simulink model "INTEGRATION_TEST_01"  (Simulink 8.1)
settings: Solver=ode4  StartTime=0.0  StopTime=inf  FixedStep=Ts  MaxStep=1e-3  RelTol=1e-3
PostLoadFcn:
  | INTEGRATION_TEST_01_init;
InitFcn:
  | INTEGRATION_TEST_01_init;
values from neighbouring files (symbols this model uses):
  CMD_signals = [1 2 3 4 5 6 7 8 9 10 11 12 ... (1568 elements, 49x32)]    [CMD_signals.mat]    (also in TestProcedure_xlsRead.m = [time_vec POI_all diesel solarIrr solarBreaker CHP load_gain)
  SIM_HIL = 0    [INTEGRATION_TEST_01_init.m]
  Ts = 100E-6    (= 0.0001)    [INTEGRATION_TEST_01_init.m]
undefined symbols (not defined in the file or in its folder): cable_spec, fdesignblkfcn, gcbh, Left, NG_CHP, NG_CHP_lib, ph, relay_par, type, V
libraries: simulink x23, rtio_opalrt_common x21, rtlab x7, powerlib_extras x7, simulink_extras x7, cables_lib x6, breaker_lib x4, rtio_generic_modbus x4, rteventslib x4, Load_lib x3, powerlib x2, ssn_lib x2
(part 3 of 3)

== matlab function SM_system/Scheduler ==
  data: u input double; y output double; CMD_signals input double; n input double; n1 output double
function [y,n1] = fcn(u,CMD_signals,n)
% Author: Matthew Backes, MIT Lincoln Laboratory
% Date: 8/16/2016
%
% Edited 9/6/2016 by E. Corbett to remove repeated Modbus register 0007 for
% DSO Import value
%
% This function takes in the test sequence signals from a .mat file which
% is generated with the ____.m script. It then updates the parameters
% within the simulink model according to the time stamp of the test
% sequence command signals.
% CMD column 1 = time
% CMD column 2 = POI feeder 1 SEL relay
% CMD column 3 = POI feeder 2 SEL relay
% CMD column 4 = POI feeder 3 SEL relay
% CMD column 5 = diesel breaker
% CMD column 6 = solar irradiance gain
% CMD column 7 = solar breaker
% CMD column 8 = CHP breaker
% CMD column 9 = load gain
% CMD column 10 = motor 1 breaker
% CMD column 11 = motor 2 breaker
% CMD column 12 = fault location 1
% CMD column 13 = fault location 2
% CMD column 14 = fault location 3
% CMD column 15 = fault location 4
% CMD column 16 = fault location 5
% CMD column 17 = fault location 6
% CMD column 18 = fault location 7
% CMD column 19 = fault location 8 SECT
%
% Next section is for dso modbus slave
% 
% CMD column 20 = dso Disconnect command
% CMD column 21 = dso Reconnect command
% CMD column 22 = dso Export command
% CMD column 23 = dso Import command
% CMD column 24 = dso power factor command
% CMD column 25 = dso VAR support command
% CMD column 26 = dso Demand Response command
% CMD column 27 = dso Import/export value
% CMD column 28 = dso power factor value
% CMD column 29 = dso VAR value
% CMD column 30 = dso DR value
% CMD column 31 = dso Command start time
% CMD column 32 = dso command duration

y = u;

coder.extrinsic('set_param') %declare set_param as an extrinsic function
coder.extrinsic('num2str') %declare num2str as an extrinsic function
%%% coder.extrinsic('tcpip')

time = CMD_signals(:,1); 
%time_lastCMD = time(length(time)); %do i need this anymore?
numCMDs = length(time);
%%% DMS_ipaddr = '192.168.10.40';
%%% DMS_ipaddr = '127.0.0.1';
%%% POI_F1_ipaddr = '192.168.10.41';
%%% POI_F2_ipaddr = '192.168.10.42';
%%% POI_F3_ipaddr = '192.168.10.43';
%%% port = 512;

%%%handles=tcpip(DMS_ipaddr, port,'Timeout',1);    %Create the tcpip object
%%%set(handles, 'InputBufferSize', 512);       %assign the buffer
%%%%set(handles, 'ByteOrder', 'bigEndian');              %specify the order in which bytes are transmitted

% set(handles, 'Connected', 0);                            %default is not connected
% try 
%%%Status=get(handles, 'Status');
%    if ~strcmp(Status,'open')       %if not open then 
%        Tcp=get(handles, 'tcp');
%%%%%%%%%%%        fopen(handles);                     %open a connection
%        set(handles, 'connected', 1);                   %connected
%    end


if n > numCMDs   %do nothing if we have exhausted all commands
    n1 = n;
else
    if u > time(n) % when the simulation time is greater than the command signal time, execute set_param
        n1 = n+1; % increment to next command to execute
        
        %parameters to set within simulink model
        set_param('INTEGRATION_TEST_01/SM_system/TestSequenceCommands','load_gain',num2str(CMD_signals(n,9)),'fault1',num2str(CMD_signals(n,12)),'fault2',num2str(CMD_signals(n,13)),'fault3',num2str(CMD_signals(n,14)),'fault4',num2str(CMD_signals(n,15)),'fault5',num2str(CMD_signals(n,16)),'fault6',num2str(CMD_signals(n,17)),'fault7',num2str(CMD_signals(n,18)),'fault8',num2str(CMD_signals(n,19))); 

        set_param('INTEGRATION_TEST_01/SM_system/DMSCommandsToMGC','DSO_Start_Time',num2str(CMD_signals(n,31)),'DSO_Duration',num2str(CMD_signals(n,32)),'DSO_Disconnect',num2str(CMD_signals(n,20)),'DSO_Export',num2str(CMD_signals(n,22)),'Import_Export_Value',num2str(CMD_signals(n,27)),'DSO_PF_Support',num2str(CMD_signals(n,24)),'PF_Value',num2str(CMD_signals(n,28)),'DSO_VAR_Support',num2str(CMD_signals(n,25)),'VAR_Value',num2str(CMD_signals(n,30)));
        
        
     else  % wait until the simulation time has eclisped the next command time
        n1 = n; 
    end
end
